simulink model "ubutest"  (R2013a)
settings: Solver=ode45  StartTime=0.0  StopTime=t_end  RelTol=1e-3
values from neighbouring files (symbols this model uses):
  Mu = (3.9856e+14)    (= 398560000000000)    [ATV_laplace_potentials_test0.m]    (also in CW_anlytical.m; Controlled_motion_test1.m; EOS_test.m; Hill_TEST.m)
  R_0c = (R_0t+rand(3,1)*0.25*1e2)    [ATV_laplace_potentials_test0.m]    (also in CW_anlytical.m = [R_C;0;0]; Controlled_motion_test1.m = (R_0t+X_obs+rand(3,1)*0.25*1e2); Hill_TEST.m = (R_0t-rand(3,1)*0.5*1e2); Hill_TEST_INTEGR.m = (R_0t-[d_TC;0;0]))
  R_0t = [R_T;0;0]    [CW_anlytical.m]    (also in Controlled_motion_test1.m = [(r_Earth+h_orb);0;0]; EOS_test.m = [(r_Earth+h_orb);0;0]; Hill_TEST.m = [(r_Earth+h_orb);0;0]; Hill_TEST_INTEGR.m = [(r_Earth+h_orb);0;0])
  V_0c = (V_0t+rand(3,1)*0.5*1e-1)    [ATV_laplace_potentials_test0.m]    (also in CW_anlytical.m = [0;sqrt(Mu/norm(R_0c));0]; Controlled_motion_test1.m = (V_0t-rand(3,1)*0.25*1e-2); Hill_TEST.m; Hill_TEST_INTEGR.m = [0;omega*R_C;0])
  V_0t = [0;sqrt(Mu/(r_Earth+h_orb));0]    [CW_anlytical.m]    (also in Controlled_motion_test1.m; EOS_test.m; Hill_TEST.m; Hill_TEST_INTEGR.m)
undefined symbols (not defined in the file or in its folder): r_0, v_0
settings Model: Creator=teo  LastModifiedBy=teo

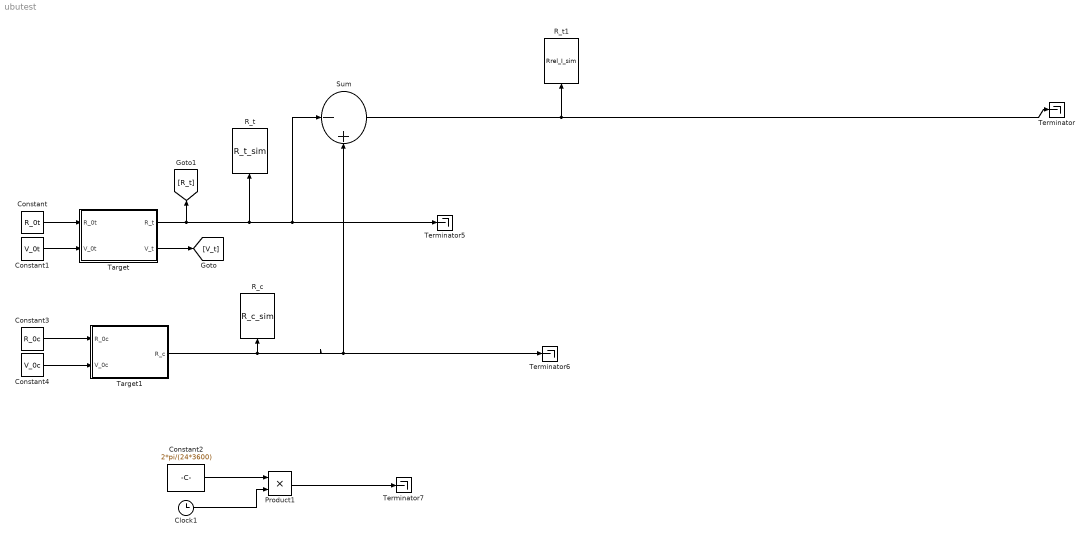
== system ubutest ==
  Clock1 : Clock
  Constant : Constant  Value=R_0t  VectorParams1D=off
  Constant1 : Constant  Value=V_0t  VectorParams1D=off
  Constant2 : Constant  Value=2*pi/(24*3600)
  Constant3 : Constant  Value=R_0c  VectorParams1D=off
  Constant4 : Constant  Value=V_0c  VectorParams1D=off
  Product1 : Product
  R_c : ToWorkspace  VariableName=R_c_sim  SampleTime=-1  SaveFormat=Structure With Time
  R_t : ToWorkspace  VariableName=R_t_sim  SampleTime=-1  SaveFormat=Structure With Time
  R_t1 : ToWorkspace  VariableName=Rrel_I_sim  SampleTime=-1  SaveFormat=Structure With Time
  Sum : Sum  Inputs=|-+
  Target : Subsystem
  Target1 : Subsystem
  Terminator{,5..7} (4 alike) : Terminator
  wires:
  Constant2/1 -> Product1/1
  Product1/1 -> Terminator7/1
  Clock1/1 -> Product1/2
  Target/1(R_t) -> [R_t], Sum/1, Terminator5/1, R_t/1
  Constant/1 -> Target/1(R_0t)
  Constant1/1 -> Target/2(V_0t)
  Target1/1(R_c) -> Sum/2, Terminator6/1, R_c/1
  Constant3/1 -> Target1/1(R_0c)
  Constant4/1 -> Target1/2(V_0c)
  Target/2("V_t ") -> [V_t]
  Sum/1 -> R_t1/1, Terminator/1

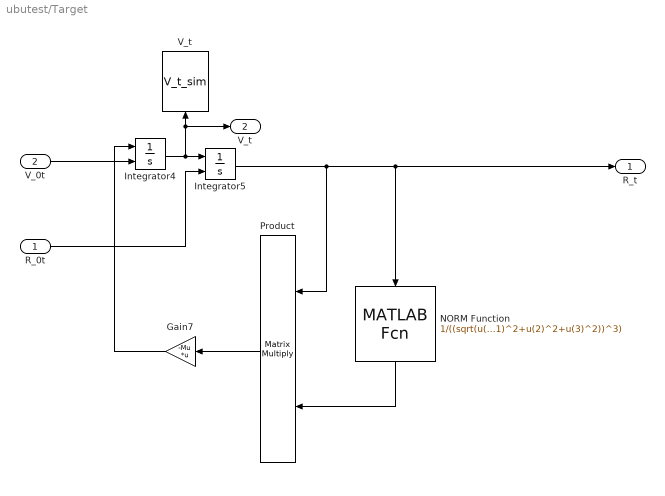
== system ubutest/Target ==
  R_0t : Inport
  V_0t : Inport  Port=2
  Gain7 : Gain  Gain=-Mu  Multiplication=Matrix(K*u)
  Integrator4 : Integrator  InitialConditionSource=external  InitialCondition=v_0
  Integrator5 : Integrator  InitialConditionSource=external  InitialCondition=r_0
  NORM Function : MATLABFcn  MATLABFcn=1/((sqrt(u(1)^2+u(2)^2+u(3)^2))^3)  OutputDimensions=1
  Product : Product  Multiplication=Matrix(*)
  V_t : ToWorkspace  VariableName=V_t_sim  SampleTime=-1  SaveFormat=Structure With Time
  R_t : Outport
  "V_t " : Outport  Port=2
  wires:
  Integrator5/1 -> R_t/1, NORM Function/1, Product/1
  Integrator4/1 -> Integrator5/1, "V_t "/1, V_t/1
  Gain7/1 -> Integrator4/1
  Product/1 -> Gain7/1
  NORM Function/1 -> Product/2
  V_0t/1 -> Integrator4/2
  R_0t/1 -> Integrator5/2

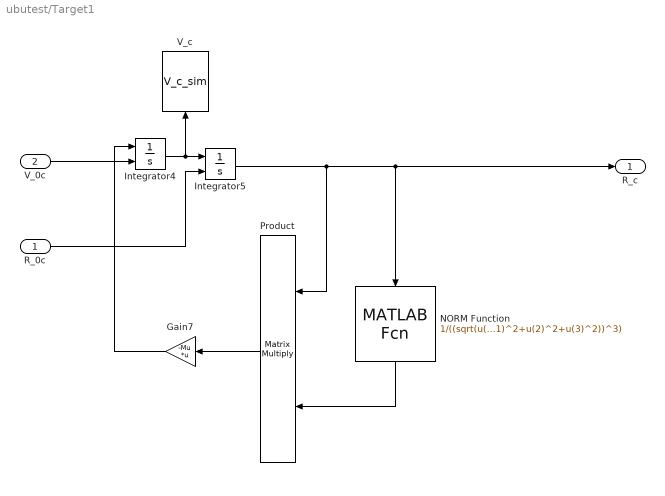
== system ubutest/Target1 ==
  R_0c : Inport
  V_0c : Inport  Port=2
  Gain7 : Gain  Gain=-Mu  Multiplication=Matrix(K*u)
  Integrator4 : Integrator  InitialConditionSource=external  InitialCondition=v_0
  Integrator5 : Integrator  InitialConditionSource=external  InitialCondition=r_0
  NORM Function : MATLABFcn  MATLABFcn=1/((sqrt(u(1)^2+u(2)^2+u(3)^2))^3)  OutputDimensions=1
  Product : Product  Multiplication=Matrix(*)
  V_c : ToWorkspace  VariableName=V_c_sim  SampleTime=-1  SaveFormat=Structure With Time
  R_c : Outport
  wires:
  Integrator5/1 -> R_c/1, NORM Function/1, Product/1
  Integrator4/1 -> Integrator5/1, V_c/1
  Gain7/1 -> Integrator4/1
  Product/1 -> Gain7/1
  NORM Function/1 -> Product/2
  V_0c/1 -> Integrator4/2
  R_0c/1 -> Integrator5/2
